simulink model "joystick_control"  (R2012b)
settings: Solver=FixedStepDiscrete  StartTime=0.0  StopTime=inf  FixedStep=0.04  RelTol=1e-3
libraries: etargetslib x14, dspnetwork x11, dspmtrx3 x7, xpcseriallib x7, visionsinks x2, simulink x2, visionstatistics x1, visiontextngfix x1, aerolibanimutils x1, SimulinkExecutionControl x1
settings Model: Creator=Ballistyx  LastModifiedBy=JLEE
settings DataIOCC: SignalLoggingSaveFormat=ModelDataLogs
settings DebuggingCC: MultiTaskDSMMsg=warning  MultiTaskCondExecSysMsg=none  FcnCallInpInsideContextMsg=EnableAllAsWarning  StrictBusMsg=None
settings SFSimCC: SFSimEnableDebug=off
settings RTWCC: IncludeERTFirstTime=on

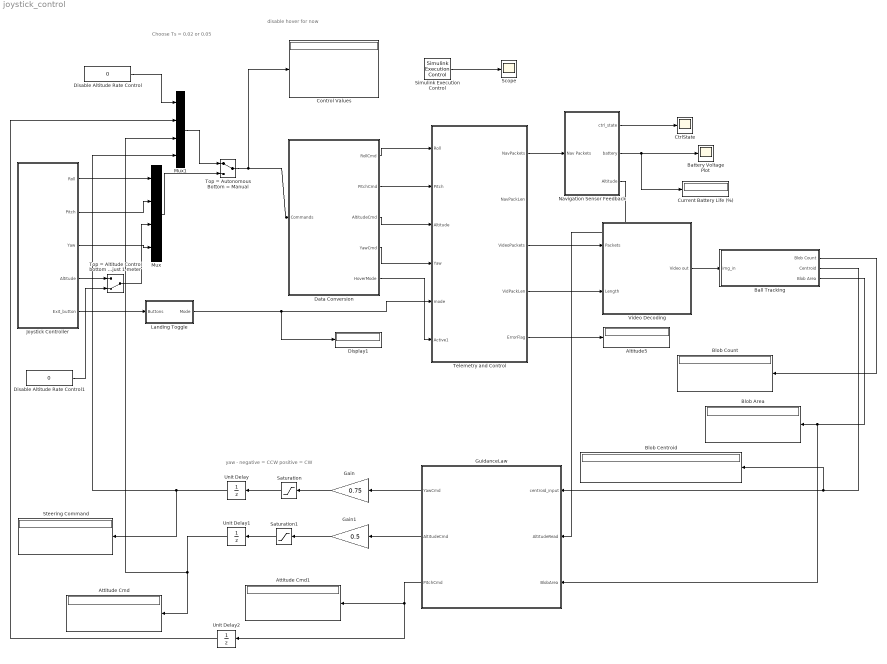
== system joystick_control ==
  note: Choose Ts = 0.02 or 0.05
  note: yaw - negative = CCW
      | positive = CW
  note: disable hover for now
  Altitude5 : Display
  Attitude Cmd : Display
  Attitude Cmd1 : Display
  Ball Tracking : Subsystem
  Battery Voltage Plot : Scope
  Blob Area : Display
  Blob Centroid : Display
  Blob Count : Display
  Control Values : Display
  CtrlState : Scope
      settings: YMin=124518  YMax=137626  SaveName=ScopeData2
  Current Battery Life (%) : Display
  Data Conversion : Subsystem
  Disable Altitude Rate Control : Constant  Value=0
  Disable Altitude Rate Control1 : Constant  Value=0
  Display1 : Display
  Gain : Gain  Gain=0.75
  Gain1 : Gain  Gain=0.5
  GuidanceLaw : Stateflow chart  TreatAsAtomicUnit=on
  Joystick Controller : Subsystem
  Landing Toggle : Subsystem
  Mux : Mux
  Mux1 : Mux
  Navigation Sensor Feedback : Subsystem
  Saturation : Saturate  UpperLimit=1  LowerLimit=-1
  Saturation1 : Saturate  UpperLimit=1  LowerLimit=-1
  Scope : Scope
  Simulink Execution Control : SimulinkExecutionControl/Simulink Execution Control  proc_pri=NORMAL_PRIORITY_CLASS  thread_pri=THREAD_PRIORITY_NORMAL  rt_sim=on  factor=1  ovrrun=Continue execution  Ts=-1
  Steering Command : Display
  Telemetry and Control : Stateflow chart  TreatAsAtomicUnit=on
  Top = Altitude Control bottom = Auto adjust 1-meter : ManualSwitch  CurrentSetting=0
  Top = Autonomous Bottom = Manual : ManualSwitch
  Unit Delay : UnitDelay  SampleTime=-1
  Unit Delay1 : UnitDelay  SampleTime=-1
  Unit Delay2 : UnitDelay  SampleTime=-1
  Video Decoding : Subsystem
  wires:
  Data Conversion/5(HoverMode) -> Telemetry and Control/6(Active1)
  Telemetry and Control/4(VidPackLen) -> Video Decoding/2(Length)
  Telemetry and Control/5(ErrorFlag) -> Altitude5/1
  Data Conversion/2(PitchCmd) -> Telemetry and Control/2(Pitch)
  Data Conversion/1(RollCmd) -> Telemetry and Control/1(Roll)
  Telemetry and Control/3(VideoPackets) -> Video Decoding/1(Packets)
  Simulink Execution Control/1 -> Scope/1
  Disable Altitude Rate Control/1 -> Mux1/1
  Landing Toggle/1(Mode) -> Telemetry and Control/5(mode), Display1/1
  Video Decoding/1(Video out) -> Ball Tracking/1(img_in)
  Ball Tracking/1(Blob Count) -> Blob Count/1
  Telemetry and Control/1(NavPackets) -> Navigation Sensor Feedback/1(Nav Packets)
  Ball Tracking/2(Centroid) -> GuidanceLaw/1(centroid_input), Blob Centroid/1
  Navigation Sensor Feedback/2(battery) -> Current Battery Life (%)/1, Battery Voltage Plot/1
  Navigation Sensor Feedback/1(ctrl_state) -> CtrlState/1
  GuidanceLaw/1(YawCmd) -> Gain/1
  Saturation/1 -> Unit Delay/1
  Unit Delay/1 -> Steering Command/1, Mux1/4
  Gain/1 -> Saturation/1
  Data Conversion/4(YawCmd) -> Telemetry and Control/4(Yaw)
  Data Conversion/3(AltitudeCmd) -> Telemetry and Control/3(Altitude)
  Joystick Controller/5(Exit_button) -> Landing Toggle/1(Buttons)
  Joystick Controller/1(Roll) -> Mux/1
  Joystick Controller/2(Pitch) -> Mux/2
  Joystick Controller/3(Yaw) -> Mux/4
  Mux1/1 -> Top = Autonomous Bottom = Manual/1
  Mux/1 -> Top = Autonomous Bottom = Manual/2
  Top = Autonomous Bottom = Manual/1 -> Data Conversion/1(Commands), Control Values/1
  Ball Tracking/3(Blob Area) -> GuidanceLaw/3(BlobArea), Blob Area/1
  Navigation Sensor Feedback/3(Altitude) -> GuidanceLaw/2(AltitudeRead)
  GuidanceLaw/2(AltitudeCmd) -> Gain1/1
  Gain1/1 -> Saturation1/1
  Unit Delay1/1 -> Mux1/3, Attitude Cmd/1
  Joystick Controller/4(Altitude) -> Top = Altitude Control bottom = Auto adjust 1-meter/1
  Top = Altitude Control bottom = Auto adjust 1-meter/1 -> Mux/3
  Disable Altitude Rate Control1/1 -> Top = Altitude Control bottom = Auto adjust 1-meter/2
  Saturation1/1 -> Unit Delay1/1
  GuidanceLaw/3(PitchCmd) -> Unit Delay2/1, Attitude Cmd1/1
  Unit Delay2/1 -> Mux1/2

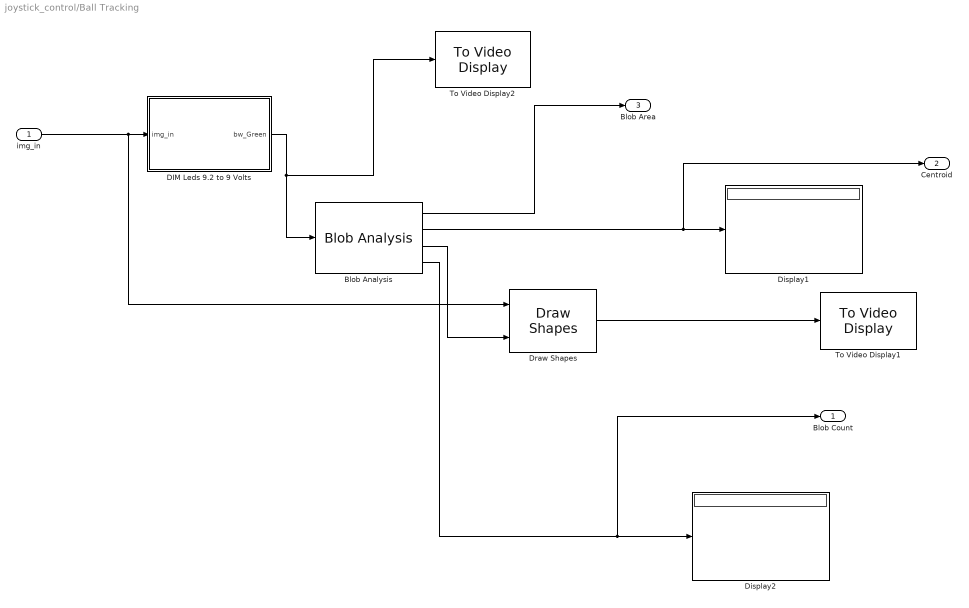
== system joystick_control/Ball Tracking ==
  img_in : Inport
  Blob Analysis : visionstatistics/Blob Analysis  Tag=vipblks_row_conv  area=on  centroid=on  bBox=on  majorAxis=off  minorAxis=off  angle=off  eccentricity=off  equivDiameterSq=off  extent=off  perimeter=off  maxBlobs=1  warnIfNumBlobsExceeded=off  isCount=on  useMinArea=on  minArea=30  useMaxArea=off  maxArea=intmax('uint32')  excludeBorderBlob=on  outDT=double  isOutVarDim=off  isFill=on  fillValues=-1  conn=8  isLabel=off  outputMode=Binary point scaling  outputWordLength=32  outputFracLength=16  firstCoeffMode=Binary point scaling  firstCoeffWordLength=16  firstCoeffFracLength=14  secondCoeffMode=Binary point scaling  secondCoeffWordLength=32  secondCoeffFracLength=16  accumMode=Binary point scaling  accumWordLength=32  accumFracLength=0  prodOutputMode=Binary point scaling  prodOutputWordLength=32  prodOutputFracLength=16  roundingMode=Floor  overflowMode=off
  DIM Leds 9.2 to 9 Volts : MATLAB Function  TreatAsAtomicUnit=on
  Display1 : Display
  Display2 : Display
  Draw Shapes : visiontextngfix/Draw Shapes  shape=Rectangles  fill=off  fillClrSource=Specify via dialog  display=White  intensity=200  color=[200 255 100]  opacity=0.6  viewport=Entire image  antialiasing=off  inType=Obsolete  imagePorts=One multidimensional signal  prodOutputMode=Binary point scaling  prodOutputWordLength=32  prodOutputFracLength=14  memoryMode=Specify word length  memoryWordLength=16  memoryFracLength=15  roundingMode=Floor  overflowMode=off
  To Video Display1 : visionsinks/To Video Display  inputType=Obsolete  imagePorts=One multidimensional signal  OutputDevice=On-screen video monitor  fullScreen=off  videoWindowX=-7  videoWindowY=-15  saveWindowSize=off  videoWindowWidth=1566  videoWindowHeight=1001  dataOrg=Column-major  openAtMdlStart=on  isWindowOpen=on  inputColorFormat=RGB
  To Video Display2 : visionsinks/To Video Display  inputType=Obsolete  imagePorts=One multidimensional signal  OutputDevice=On-screen video monitor  fullScreen=off  videoWindowX=420  videoWindowY=155  saveWindowSize=off  videoWindowWidth=320  videoWindowHeight=240  dataOrg=Column-major  openAtMdlStart=on  isWindowOpen=on  inputColorFormat=RGB
  Blob Count : Outport
  Centroid : Outport  Port=2
  Blob Area : Outport  Port=3
  wires:
  img_in/1 -> DIM Leds 9.2 to 9 Volts/1(img_in), Draw Shapes/1
  DIM Leds 9.2 to 9 Volts/1(bw_Green) -> Blob Analysis/1, To Video Display2/1
  Blob Analysis/3 -> Draw Shapes/2
  Draw Shapes/1 -> To Video Display1/1
  Blob Analysis/2 -> Display1/1, Centroid/1
  Blob Analysis/4 -> Display2/1, Blob Count/1
  Blob Analysis/1 -> Blob Area/1

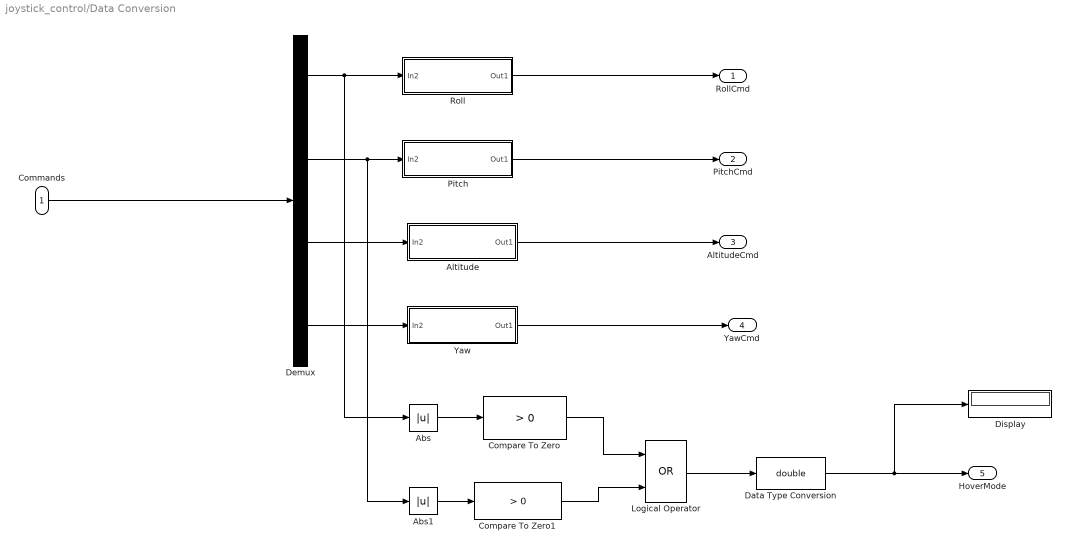
== system joystick_control/Data Conversion ==
  Commands : Inport
  Abs : Abs
  Abs1 : Abs
  Altitude : Subsystem
  Compare To Zero : simulink/Logic and Bit Operations/Compare To Zero  relop=>  OutDataTypeStr=uint8
  Compare To Zero1 : simulink/Logic and Bit Operations/Compare To Zero  relop=>  OutDataTypeStr=uint8
  Data Type Conversion : DataTypeConversion  OutDataTypeStr=double
  Demux : Demux
  Display : Display
  Logical Operator : Logic  Operator=OR  AllPortsSameDT=off  OutDataTypeStr=boolean
  Pitch : Subsystem
  Roll : Subsystem
  Yaw : Subsystem
  RollCmd : Outport
  PitchCmd : Outport  Port=2
  AltitudeCmd : Outport  Port=3
  YawCmd : Outport  Port=4
  HoverMode : Outport  Port=5
  wires:
  Demux/1 -> Roll/1(In2), Abs/1
  Demux/2 -> Pitch/1(In2), Abs1/1
  Demux/3 -> Altitude/1(In2)
  Demux/4 -> Yaw/1(In2)
  Commands/1 -> Demux/1
  Roll/1(Out1) -> RollCmd/1
  Pitch/1(Out1) -> PitchCmd/1
  Altitude/1(Out1) -> AltitudeCmd/1
  Yaw/1(Out1) -> YawCmd/1
  Compare To Zero/1 -> Logical Operator/1
  Compare To Zero1/1 -> Logical Operator/2
  Logical Operator/1 -> Data Type Conversion/1
  Data Type Conversion/1 -> HoverMode/1, Display/1
  Abs/1 -> Compare To Zero/1
  Abs1/1 -> Compare To Zero1/1

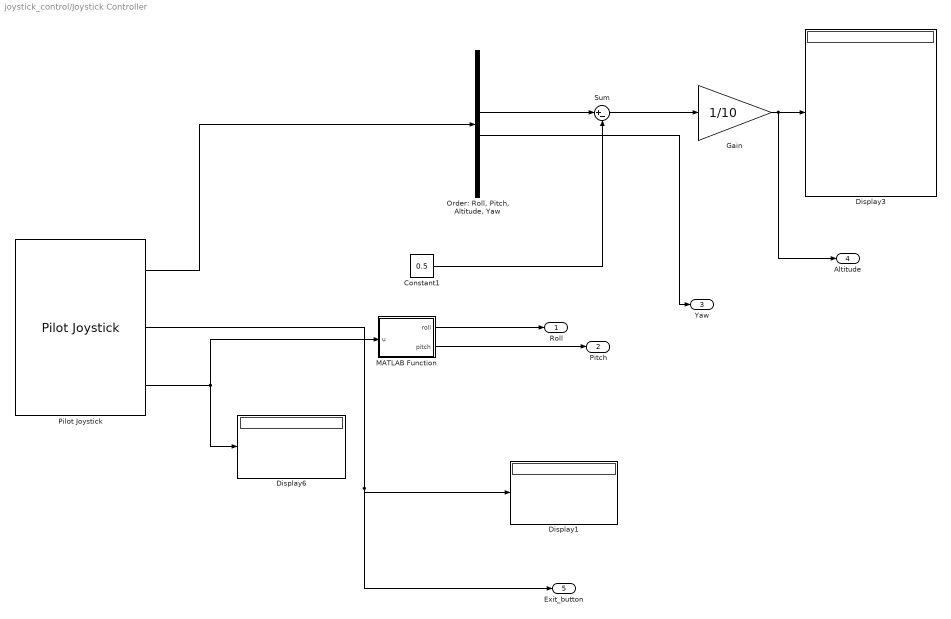
== system joystick_control/Joystick Controller ==
  Constant1 : Constant  Value=0.5
  Display1 : Display
  Display3 : Display
  Display6 : Display
  Gain : Gain  Gain=1/10
  MATLAB Function : MATLAB Function  TreatAsAtomicUnit=on
  "Order: Roll, Pitch, Altitude, Yaw" : Demux  Outputs=6
  Pilot Joystick : aerolibanimutils/Pilot Joystick  JoystickID=Joystick1  OutputConfiguration=AllOutputs  SampleTime=-1
  Sum : Sum  Inputs=|+-
  Roll : Outport
  Pitch : Outport  Port=2
  Yaw : Outport  Port=3
  Altitude : Outport  Port=4
  Exit_button : Outport  Port=5
  wires:
  Pilot Joystick/1 -> "Order: Roll, Pitch, Altitude, Yaw"/1
  Pilot Joystick/3 -> Display6/1, MATLAB Function/1(u)
  "Order: Roll, Pitch, Altitude, Yaw"/3 -> Sum/1
  Constant1/1 -> Sum/2
  Sum/1 -> Gain/1
  MATLAB Function/1(roll) -> Roll/1
  MATLAB Function/2(pitch) -> Pitch/1
  Gain/1 -> Display3/1, Altitude/1
  "Order: Roll, Pitch, Altitude, Yaw"/4 -> Yaw/1
  Pilot Joystick/2 -> Display1/1, Exit_button/1

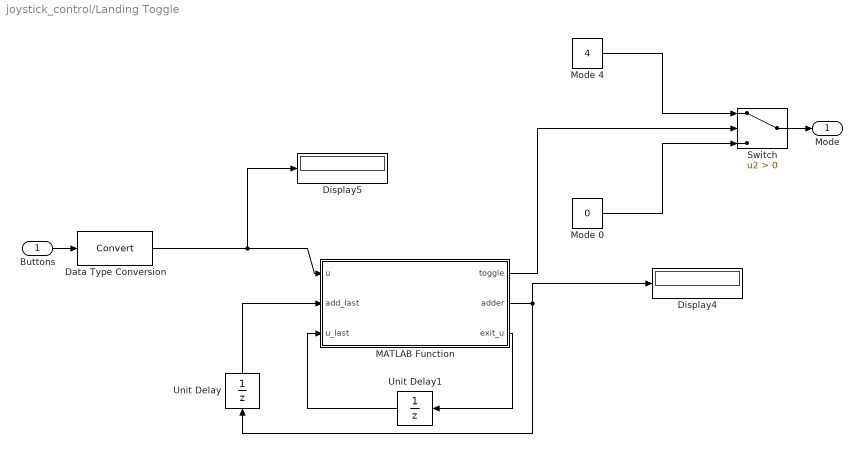
== system joystick_control/Landing Toggle ==
  Buttons : Inport
  Data Type Conversion : DataTypeConversion
  Display4 : Display
  Display5 : Display
  MATLAB Function : MATLAB Function  TreatAsAtomicUnit=on
  Mode 0 : Constant  Value=0
  Mode 4 : Constant  Value=4
  Switch : Switch  Criteria=u2 > Threshold
  Unit Delay : UnitDelay  SampleTime=-1
  Unit Delay1 : UnitDelay  SampleTime=-1
  Mode : Outport
  wires:
  Unit Delay/1 -> MATLAB Function/2(add_last)
  MATLAB Function/2(adder) -> Display4/1, Unit Delay/1
  MATLAB Function/3(exit_u) -> Unit Delay1/1
  Unit Delay1/1 -> MATLAB Function/3(u_last)
  Data Type Conversion/1 -> MATLAB Function/1(u), Display5/1
  MATLAB Function/1(toggle) -> Switch/2
  Mode 4/1 -> Switch/1
  Mode 0/1 -> Switch/3
  Switch/1 -> Mode/1
  Buttons/1 -> Data Type Conversion/1

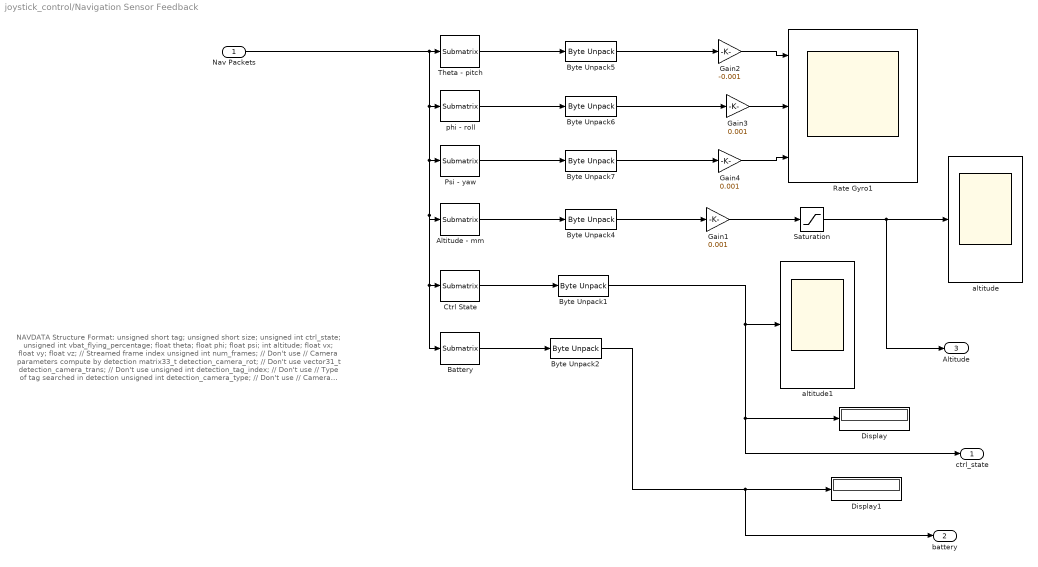
== system joystick_control/Navigation Sensor Feedback ==
  note: NAVDATA Structure Format:
      |
      |         unsigned short tag;
      |         unsigned short size;
      |         unsigned int   ctrl_state;
      |         unsigned int   vbat_flying_percentage;
      |         float          theta;
      |         float          phi;
      |         float          psi;
      |         int            altitude;
      |         float          vx;
      |         float          vy;
      |         float          vz;
      |
      |         // Streamed frame index
      |         unsigned int num_frames;                // Don't use
      |
      |         // Camera parameters compute by detection
      |         matrix33_t   detection_camera_rot;      // Don't use
      |         vector31_t   detection_camera_trans;    // Don't use
      |         unsigned int detection_tag_index;       // Don't use
      |
      |         // Type of tag searched in detection
      |         unsigned int detection_camera_type;     // Don't use
      |
      |         // Camera parameters compute by drone
      |         matrix33_t drone_camera_rot;            // Don't use
      |         vector31_t drone_camera_trans;          // Don't use
  Nav Packets : Inport
  Altitude - mm : dspmtrx3/Submatrix  RowSpan=Range of rows  RowStartMode=Index  RowStartIndex=41  RowEndMode=Index  RowEndIndex=44  ColSpan=All columns  ColStartMode=Index  ColStartIndex=4  ColEndMode=Index  ColEndIndex=4
  Battery : dspmtrx3/Submatrix  RowSpan=Range of rows  RowStartMode=Index  RowStartIndex=25  RowEndMode=Index  RowEndIndex=28  ColSpan=All columns  ColStartMode=Index  ColStartIndex=4  ColEndMode=Index  ColEndIndex=4
  Byte Unpack1 : etargetslib/Byte Unpack  dimensions={[1]}  datatypes={'uint32'}  byteAlign=1
  Byte Unpack2 : etargetslib/Byte Unpack  dimensions={[1]}  datatypes={'uint32'}  byteAlign=1
  Byte Unpack4 : etargetslib/Byte Unpack  dimensions={[1]}  datatypes={'uint32'}  byteAlign=1
  Byte Unpack5 : etargetslib/Byte Unpack  dimensions={[1]}  datatypes={'single'}  byteAlign=1
  Byte Unpack6 : etargetslib/Byte Unpack  dimensions={[1]}  datatypes={'single'}  byteAlign=1
  Byte Unpack7 : etargetslib/Byte Unpack  dimensions={[1]}  datatypes={'single'}  byteAlign=1
  Ctrl State : dspmtrx3/Submatrix  RowSpan=Range of rows  RowStartMode=Index  RowStartIndex=21  RowEndMode=Index  RowEndIndex=24  ColSpan=All columns  ColStartMode=Index  ColStartIndex=4  ColEndMode=Index  ColEndIndex=4
  Display : Display
  Display1 : Display
  Gain1 : Gain  Gain=0.001  OutDataTypeStr=double
  Gain2 : Gain  Gain=-0.001
  Gain3 : Gain  Gain=0.001
  Gain4 : Gain  Gain=0.001
  Psi - yaw : dspmtrx3/Submatrix  RowSpan=Range of rows  RowStartMode=Index  RowStartIndex=37  RowEndMode=Index  RowEndIndex=40  ColSpan=All columns  ColStartMode=Index  ColStartIndex=4  ColEndMode=Index  ColEndIndex=4
  Rate Gyro1 : Scope  NumInputPorts=3
      settings: TimeRange=18  YMin=-0.75~2.935~53.5  YMax=0~3~60  SaveName=NavData_Simulink1
  Saturation : Saturate  UpperLimit=10  LowerLimit=0  OutDataTypeStr=Inherit: Inherit via back propagation
  Theta - pitch : dspmtrx3/Submatrix  RowSpan=Range of rows  RowStartMode=Index  RowStartIndex=29  RowEndMode=Index  RowEndIndex=32  ColSpan=All columns  ColStartMode=Index  ColStartIndex=4  ColEndMode=Index  ColEndIndex=4
  altitude : Scope
      settings: YMin=0.242  YMax=0.24305  SaveName=NavData_Simulink
  altitude1 : Scope
      settings: YMin=0.242  YMax=0.24305  SaveName=NavData_Simulink2
  phi - roll : dspmtrx3/Submatrix  RowSpan=Range of rows  RowStartMode=Index  RowStartIndex=33  RowEndMode=Index  RowEndIndex=36  ColSpan=All columns  ColStartMode=Index  ColStartIndex=4  ColEndMode=Index  ColEndIndex=4
  ctrl_state : Outport
  battery : Outport  Port=2
  Altitude : Outport  Port=3
  wires:
  Altitude - mm/1 -> Byte Unpack4/1
  Theta - pitch/1 -> Byte Unpack5/1
  phi - roll/1 -> Byte Unpack6/1
  Psi - yaw/1 -> Byte Unpack7/1
  Byte Unpack5/1 -> Gain2/1
  Byte Unpack6/1 -> Gain3/1
  Byte Unpack7/1 -> Gain4/1
  Byte Unpack4/1 -> Gain1/1
  Gain1/1 -> Saturation/1
  Gain2/1 -> Rate Gyro1/1
  Gain3/1 -> Rate Gyro1/2
  Gain4/1 -> Rate Gyro1/3
  Nav Packets/1 -> Psi - yaw/1, Altitude - mm/1, Ctrl State/1, Battery/1, phi - roll/1, Theta - pitch/1
  Saturation/1 -> altitude/1, Altitude/1
  Ctrl State/1 -> Byte Unpack1/1
  Byte Unpack1/1 -> altitude1/1, Display/1, ctrl_state/1
  Battery/1 -> Byte Unpack2/1
  Byte Unpack2/1 -> Display1/1, battery/1

== system joystick_control/Telemetry and Control/SetVideo ==
  DataStamp : Inport
  f : TriggerPort  TriggerType=function-call
      settings: CopyFcn=Stateflow.SLINSF.SimulinkMan.removeBlockPreDeleteFcn  PreDeleteFcn=Stateflow.SLINSF.SimulinkMan.unsafePredeleteFcn
  ASCII Encode 1 : xpcseriallib/ASCII Encode   format="AT*CONFIG=%d,\\\"video:video_channel\\\",\\\"0\\\"\\r"  nvars=1  maxlength=44  vartypes={ 'uint32' }
  UDP Send : dspnetwork/UDP Send  remoteURL='192.168.1.1'  remotePort=5556  localURL='0.0.0.0'  localPortSource=Specify via dialog  localPort=5556  sampletime=-1  separateLengthPort=0
  wires:
  DataStamp/1 -> ASCII Encode 1/1
  ASCII Encode 1/1 -> UDP Send/1

== system joystick_control/Telemetry and Control/StartNavDemo ==
  note: Enable navdatademo
  DataStamp : Inport
  f : TriggerPort  TriggerType=function-call
      settings: CopyFcn=Stateflow.SLINSF.SimulinkMan.removeBlockPreDeleteFcn  PreDeleteFcn=Stateflow.SLINSF.SimulinkMan.unsafePredeleteFcn
  ASCII Encode 2 : xpcseriallib/ASCII Encode   format="AT*CONFIG=%d,\\\"general:navdata_demo\\\",\\\"TRUE\\\"\\r"  nvars=1  maxlength=43  vartypes={ 'uint32' }
  UDP Send1 : dspnetwork/UDP Send  remoteURL='192.168.1.1'  remotePort=5556  localURL='0.0.0.0'  localPortSource=Specify via dialog  localPort=5556  sampletime=-1  separateLengthPort=0
  wires:
  DataStamp/1 -> ASCII Encode 2/1
  ASCII Encode 2/1 -> UDP Send1/1

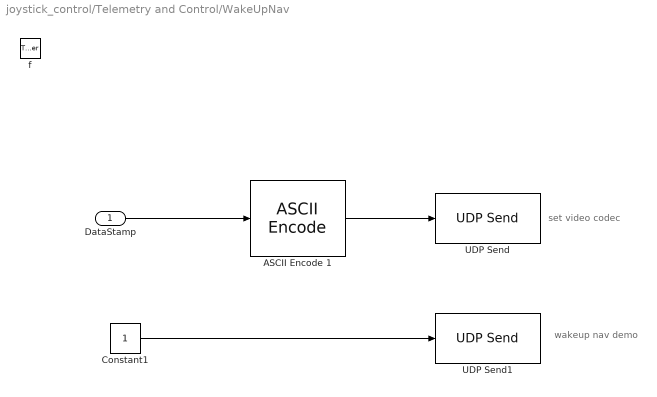
== system joystick_control/Telemetry and Control/WakeUpNav ==
  note: set video codec
  note: wakeup nav demo
  DataStamp : Inport
  f : TriggerPort  TriggerType=function-call
      settings: CopyFcn=Stateflow.SLINSF.SimulinkMan.removeBlockPreDeleteFcn  PreDeleteFcn=Stateflow.SLINSF.SimulinkMan.unsafePredeleteFcn
  ASCII Encode 1 : xpcseriallib/ASCII Encode   format="AT*CONFIG=%d,\\\"video:video_codec\\\",\\\"32\\\"\\r"  nvars=1  maxlength=44  vartypes={ 'uint32' }
  Constant1 : Constant  OutDataTypeStr=uint8  SampleTime=-1
  UDP Send : dspnetwork/UDP Send  remoteURL='192.168.1.1'  remotePort=5556  localURL='0.0.0.0'  localPortSource=Specify via dialog  localPort=5556  sampletime=-1  separateLengthPort=0
  UDP Send1 : dspnetwork/UDP Send  remoteURL='192.168.1.1'  remotePort=5554  localURL='0.0.0.0'  localPortSource=Specify via dialog  localPort=5554  sampletime=-1  separateLengthPort=0
  wires:
  DataStamp/1 -> ASCII Encode 1/1
  Constant1/1 -> UDP Send1/1
  ASCII Encode 1/1 -> UDP Send/1

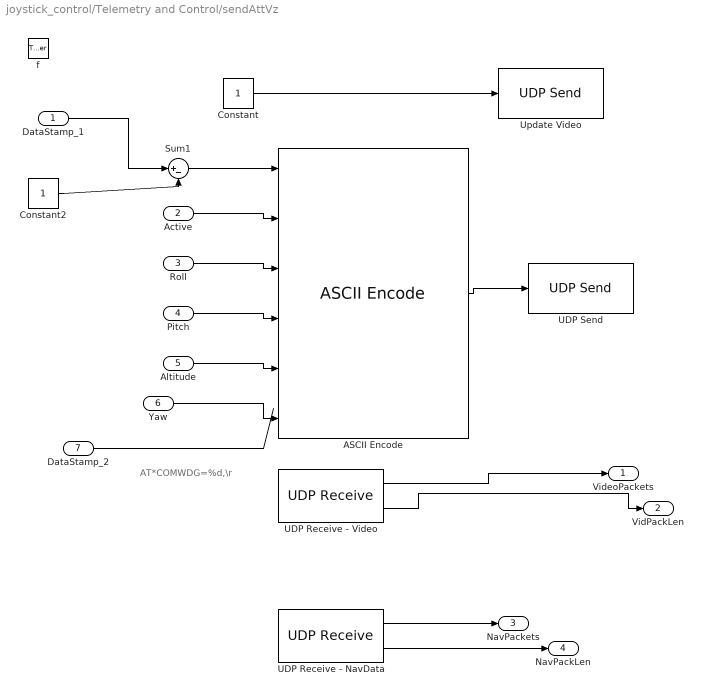
== system joystick_control/Telemetry and Control/sendAttVz ==
  note: AT*COMWDG=%d,\r
  DataStamp_1 : Inport
  Active : Inport  Port=2
  Roll : Inport  Port=3
  Pitch : Inport  Port=4
  Altitude : Inport  Port=5
  Yaw : Inport  Port=6
  DataStamp_2 : Inport  Port=7
  f : TriggerPort  TriggerType=function-call
      settings: CopyFcn=Stateflow.SLINSF.SimulinkMan.removeBlockPreDeleteFcn  PreDeleteFcn=Stateflow.SLINSF.SimulinkMan.unsafePredeleteFcn
  "ASCII Encode " : xpcseriallib/ASCII Encode   format=AT*PCMD=%d,%d,%d,%d,%d,%d\r  nvars=6  maxlength=128  vartypes={ 'double' }
  Constant : Constant  Priority=12  OutDataTypeStr=uint8  SampleTime=-1
  Constant2 : Constant
  Sum1 : Sum  Inputs=|+-
  UDP Receive - NavData : dspnetwork/UDP Receive  Priority=15  localURL='0.0.0.0'  localPort=5554  remoteURL='192.168.1.1'  remotePort=-1  recvBufferSize=500  dims=500  signalDatatype=uint8  isVarSize=off  showBlockingTime=off  blockingTime=0  sampletime=-1
  UDP Receive - Video : dspnetwork/UDP Receive  Priority=16  localURL='0.0.0.0'  localPort=5555  remoteURL='192.168.1.1'  remotePort=-1  recvBufferSize=40000*2  dims=40000  signalDatatype=uint8  isVarSize=off  showBlockingTime=off  blockingTime=0  sampletime=-1
  UDP Send : dspnetwork/UDP Send  Priority=11  remoteURL='192.168.1.1'  remotePort=5556  localURL='0.0.0.0'  localPortSource=Specify via dialog  localPort=5556  sampletime=-1  separateLengthPort=0
  Update Video : dspnetwork/UDP Send  Priority=10  remoteURL='192.168.1.1'  remotePort=5555  localURL='0.0.0.0'  localPortSource=Specify via dialog  localPort=5555  sampletime=-1  separateLengthPort=0
  VideoPackets : Outport
  VidPackLen : Outport  Port=2  OutDataTypeStr=uint16
  NavPackets : Outport  Port=3
  NavPackLen : Outport  Port=4
  wires:
  Active/1 -> "ASCII Encode "/2
  Roll/1 -> "ASCII Encode "/3
  Pitch/1 -> "ASCII Encode "/4
  Altitude/1 -> "ASCII Encode "/5
  Yaw/1 -> "ASCII Encode "/6
  DataStamp_2/1 -> ?
  DataStamp_1/1 -> Sum1/1
  Sum1/1 -> "ASCII Encode "/1
  Constant2/1 -> Sum1/2
  "ASCII Encode "/1 -> UDP Send/1
  Constant/1 -> Update Video/1
  UDP Receive - Video/2 -> VidPackLen/1
  UDP Receive - NavData/2 -> NavPackLen/1
  UDP Receive - Video/1 -> VideoPackets/1
  UDP Receive - NavData/1 -> NavPackets/1

== system joystick_control/Telemetry and Control/sendLand ==
  In1 : Inport
  f : TriggerPort  TriggerType=function-call
      settings: CopyFcn=Stateflow.SLINSF.SimulinkMan.removeBlockPreDeleteFcn  PreDeleteFcn=Stateflow.SLINSF.SimulinkMan.unsafePredeleteFcn
  "ASCII Encode " : xpcseriallib/ASCII Encode   format=AT*REF=%d,290717696\r  nvars=1  maxlength=128  vartypes={ 'double' }
  UDP Send : dspnetwork/UDP Send  remoteURL='192.168.1.1'  remotePort=5556  localURL='0.0.0.0'  localPortSource=Specify via dialog  localPort=5556  sampletime=-1  separateLengthPort=0
  wires:
  "ASCII Encode "/1 -> UDP Send/1
  In1/1 -> "ASCII Encode "/1

== system joystick_control/Telemetry and Control/sendTrim ==
  DataStamp : Inport
  f : TriggerPort  TriggerType=function-call
      settings: CopyFcn=Stateflow.SLINSF.SimulinkMan.removeBlockPreDeleteFcn  PreDeleteFcn=Stateflow.SLINSF.SimulinkMan.unsafePredeleteFcn
  "ASCII Encode " : xpcseriallib/ASCII Encode   format=AT*FTRIM=%d,\r  nvars=1  maxlength=128  vartypes={ 'double' }
  UDP Send : dspnetwork/UDP Send  remoteURL='192.168.1.1'  remotePort=5556  localURL='0.0.0.0'  localPortSource=Specify via dialog  localPort=5556  sampletime=-1  separateLengthPort=0
  wires:
  DataStamp/1 -> "ASCII Encode "/1
  "ASCII Encode "/1 -> UDP Send/1

== system joystick_control/Telemetry and Control/startHover ==
  note: disable hover for now
  DataStamp : Inport
  f : TriggerPort  TriggerType=function-call
      settings: CopyFcn=Stateflow.SLINSF.SimulinkMan.removeBlockPreDeleteFcn  PreDeleteFcn=Stateflow.SLINSF.SimulinkMan.unsafePredeleteFcn
  "ASCII Encode " : xpcseriallib/ASCII Encode   format=AT*REF=%d,290718208\r  nvars=1  maxlength=128  vartypes={ 'double' }
  UDP Send : dspnetwork/UDP Send  remoteURL='192.168.1.1'  remotePort=5556  localURL='0.0.0.0'  localPortSource=Specify via dialog  localPort=5556  sampletime=-1  separateLengthPort=0
  wires:
  DataStamp/1 -> "ASCII Encode "/1
  "ASCII Encode "/1 -> UDP Send/1

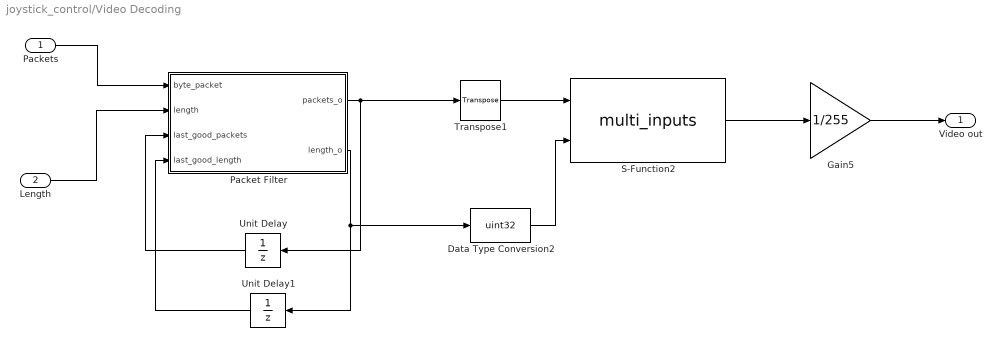
== system joystick_control/Video Decoding ==
  Packets : Inport
  Length : Inport  Port=2
  Data Type Conversion2 : DataTypeConversion  OutDataTypeStr=uint32
  Gain5 : Gain  Gain=1/255
  Packet Filter : MATLAB Function  TreatAsAtomicUnit=on
  S-Function2 : S-Function  FunctionName=multi_inputs  EnableBusSupport=off
  Transpose1 : dspmtrx3/Transpose  Hermitian=off  overflowFlag=off
  Unit Delay : UnitDelay  SampleTime=-1
  Unit Delay1 : UnitDelay  SampleTime=-1
  Video out : Outport
  wires:
  Data Type Conversion2/1 -> S-Function2/2
  S-Function2/1 -> Gain5/1
  Transpose1/1 -> S-Function2/1
  Packet Filter/1(packets_o) -> Unit Delay/1, Transpose1/1
  Unit Delay/1 -> Packet Filter/3(last_good_packets)
  Packet Filter/2(length_o) -> Unit Delay1/1, Data Type Conversion2/1
  Unit Delay1/1 -> Packet Filter/4(last_good_length)
  Packets/1 -> Packet Filter/1(byte_packet)
  Length/1 -> Packet Filter/2(length)
  Gain5/1 -> Video out/1

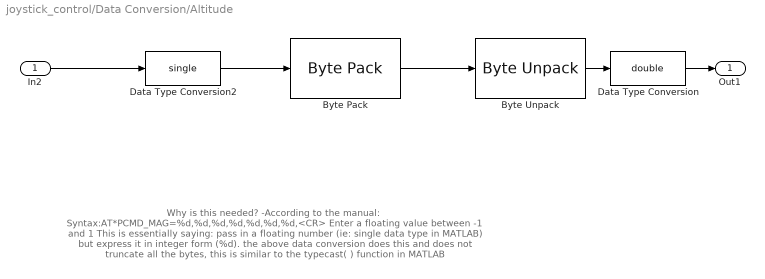
== system joystick_control/Data Conversion/Altitude ==
  note: Why is this needed?
      | -According to the manual:
      |
      | Syntax:AT*PCMD_MAG=%d,%d,%d,%d,%d,%d,%d,<CR>
      | Enter a floating value between -1 and 1
      |
      | This is essentially saying: pass in a floating number (ie: single data type in MATLAB) but express it in integer form (%d).
      | the above data conversion does this and does not truncate all the bytes, this is similar to the typecast( ) function in MATLAB
  In2 : Inport
  Byte Pack : etargetslib/Byte Pack  datatypes={'single'}  byteAlign=1
  Byte Unpack : etargetslib/Byte Unpack  dimensions={[1]}  datatypes={'int32'}  byteAlign=1
  Data Type Conversion : DataTypeConversion  OutDataTypeStr=double
  Data Type Conversion2 : DataTypeConversion  OutDataTypeStr=single
  Out1 : Outport
  wires:
  Byte Pack/1 -> Byte Unpack/1
  Byte Unpack/1 -> Data Type Conversion/1
  In2/1 -> Data Type Conversion2/1
  Data Type Conversion2/1 -> Byte Pack/1
  Data Type Conversion/1 -> Out1/1

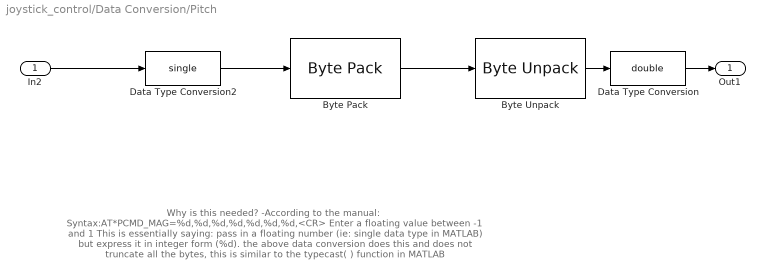
== system joystick_control/Data Conversion/Pitch ==
  note: Why is this needed?
      | -According to the manual:
      |
      | Syntax:AT*PCMD_MAG=%d,%d,%d,%d,%d,%d,%d,<CR>
      | Enter a floating value between -1 and 1
      |
      | This is essentially saying: pass in a floating number (ie: single data type in MATLAB) but express it in integer form (%d).
      | the above data conversion does this and does not truncate all the bytes, this is similar to the typecast( ) function in MATLAB
  In2 : Inport
  Byte Pack : etargetslib/Byte Pack  datatypes={'single'}  byteAlign=1
  Byte Unpack : etargetslib/Byte Unpack  dimensions={[1]}  datatypes={'int32'}  byteAlign=1
  Data Type Conversion : DataTypeConversion  OutDataTypeStr=double
  Data Type Conversion2 : DataTypeConversion  OutDataTypeStr=single
  Out1 : Outport
  wires:
  Byte Pack/1 -> Byte Unpack/1
  Byte Unpack/1 -> Data Type Conversion/1
  In2/1 -> Data Type Conversion2/1
  Data Type Conversion2/1 -> Byte Pack/1
  Data Type Conversion/1 -> Out1/1

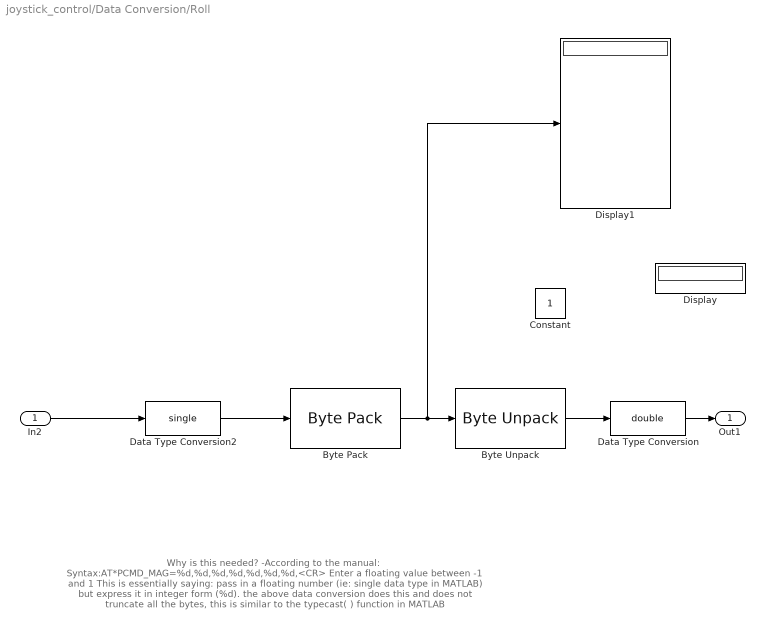
== system joystick_control/Data Conversion/Roll ==
  note: Why is this needed?
      | -According to the manual:
      |
      | Syntax:AT*PCMD_MAG=%d,%d,%d,%d,%d,%d,%d,<CR>
      | Enter a floating value between -1 and 1
      |
      | This is essentially saying: pass in a floating number (ie: single data type in MATLAB) but express it in integer form (%d).
      | the above data conversion does this and does not truncate all the bytes, this is similar to the typecast( ) function in MATLAB
  In2 : Inport
  Byte Pack : etargetslib/Byte Pack  datatypes={'single'}  byteAlign=1
  Byte Unpack : etargetslib/Byte Unpack  dimensions={[1]}  datatypes={'int32'}  byteAlign=1
  Constant : Constant
  Data Type Conversion : DataTypeConversion  OutDataTypeStr=double
  Data Type Conversion2 : DataTypeConversion  OutDataTypeStr=single
  Display : Display
  Display1 : Display
  Out1 : Outport
  wires:
  In2/1 -> Data Type Conversion2/1
  Data Type Conversion2/1 -> Byte Pack/1
  Data Type Conversion/1 -> Out1/1
  Byte Pack/1 -> Byte Unpack/1, Display1/1
  Byte Unpack/1 -> Data Type Conversion/1
  ? -> Display/1

== system joystick_control/Data Conversion/Yaw ==
  note: Why is this needed?
      | -According to the manual:
      |
      | Syntax:AT*PCMD_MAG=%d,%d,%d,%d,%d,%d,%d,<CR>
      | Enter a floating value between -1 and 1
      |
      | This is essentially saying: pass in a floating number (ie: single data type in MATLAB) but express it in integer form (%d).
      | the above data conversion does this and does not truncate all the bytes, this is similar to the typecast( ) function in MATLAB
  In2 : Inport
  Byte Pack : etargetslib/Byte Pack  datatypes={'single'}  byteAlign=1
  Byte Unpack : etargetslib/Byte Unpack  dimensions={[1]}  datatypes={'int32'}  byteAlign=1
  Data Type Conversion : DataTypeConversion  OutDataTypeStr=double
  Data Type Conversion2 : DataTypeConversion  OutDataTypeStr=single
  Out1 : Outport
  wires:
  Byte Pack/1 -> Byte Unpack/1
  Byte Unpack/1 -> Data Type Conversion/1
  In2/1 -> Data Type Conversion2/1
  Data Type Conversion2/1 -> Byte Pack/1
  Data Type Conversion/1 -> Out1/1

== matlab function joystick_control/Video Decoding/Packet Filter ==
  data: byte_packet input; packets_o output; length input uint16; last_good_packets input; length_o output uint16; last_good_length input
function [packets_o,length_o] = fcn(byte_packet,length,last_good_packets,last_good_length)
%#codegen

if length == 0
    packets_o = last_good_packets;
    length_o = last_good_length;
else
    packets_o = byte_packet; 
    length_o = length;
end

== matlab function joystick_control/Landing Toggle/MATLAB Function ==
  data: toggle output; u input; add_last input; adder output; exit_u output double; u_last input
function [toggle,adder,exit_u] = fcn(u,add_last,u_last)
%#codegen

% if u ~= last_u
% y = 1;
% else
% y = 0;    
% end
% 

if (u==64 & (u_last == 0))
    
   adder = add_last + 1;
%     exit_u = u;
else
    adder = add_last;
%     exit_u = u;
end

 exit_u = u;
 
 toggle=mod(adder,2);

% y = u;

== stateflow chart joystick_control/GuidanceLaw ==
  state Steering_Law [parallel]
    settings: executionOrder=1
    state NoBall
      YawCmd = 0;
    state WithinFOV_x
      YawCmd = 0;
    state Steering
      du: YawCmd = SteerYaw(centroid_input);
    (default) -> (junction 131)
    (junction 131) -> Steering_Law.NoBall : {i=0;
        | InitiateVariables_x();}
    Steering -> Steering_Law.NoBall [order 2] : [centroid_input[0] == -1 ]
    Steering_Law.NoBall -> WithinFOV_x : [centroid_input[0] != -1  ]
        | {i = i + 1;}
    WithinFOV_x -> Steering [order 1] : [ (centroid_input[0]<SearchField_left || centroid_input[0]>SearchField_right) && centroid_input[0] != -1]
        | {i = i + 1;}
    WithinFOV_x -> Steering_Law.NoBall [order 2] : [centroid_input[0] == -1 ]
        | {i = i + 1;}
    Steering -> WithinFOV_x [order 1] : [ (centroid_input[0]>=SearchField_left && centroid_input[0]<=SearchField_right) && centroid_input[0] != -1]
        | {i = i + 1;}
  state Pitch_Cmd [parallel]
    settings: executionOrder=3
    state NoBall
      PitchCmd = 0;
    state StopFollowing
      PitchCmd = 0;
    state FollowBall
      PitchCmd = -0.05;
    (default) -> (junction 183)
    (junction 183) -> Pitch_Cmd.NoBall : {i=0;
        | PitchInitiate();}
    StopFollowing -> Pitch_Cmd.NoBall [order 1] : [BlobArea == -1]
    Pitch_Cmd.NoBall -> StopFollowing : [BlobArea != -1]
    FollowBall -> StopFollowing : [BlobArea>BlobAreaThresholdLo || YawCmd!=0  || YawCmd!=0]
    StopFollowing -> FollowBall [order 2] : [BlobArea<=BlobAreaThresholdLo && YawCmd==0 && AltitudeCmd==0]
  state Altitude_Cmd [parallel]
    settings: executionOrder=2
    state NoBall
      AltitudeCmd  = 0;
    state WithinFOV_y
      AltitudeCmd = 0;
    state Altitude_Correct
      du: AltitudeCmd = ChangeAltitude(centroid_input);
    (default) -> (junction 158)
    (junction 158) -> Altitude_Cmd.NoBall : {i=0;
        | InitiateVariables_y();}
    Altitude_Correct -> Altitude_Cmd.NoBall [order 1] : [centroid_input[1] == -1 ]
    WithinFOV_y -> Altitude_Correct [order 2] : [ (centroid_input[1]>=SearchField_Bottom || centroid_input[1]<=SearchField_Top) && centroid_input[1] != -1]
        | {i = i + 1;}
    Altitude_Cmd.NoBall -> WithinFOV_y : [centroid_input[1] != -1  ]
        | {i = i + 1;}
    WithinFOV_y -> Altitude_Cmd.NoBall [order 1] : [centroid_input[1] == -1  ]
        | {i = i + 1;}
    Altitude_Correct -> WithinFOV_y [order 2] : [ (centroid_input[1]<SearchField_Bottom && centroid_input[1]>SearchField_Top) && centroid_input[1] != -1]
        | {i = i + 1;}
  data: YawCmd function_output double size=1; centroid_input function_input double size=2; AltitudeCmd function_output double size=1; centroid function_input double size=2; centroid_input input double size=2; Roll local double; Pitch local double; YawCmd output double =0; AltitudeRead input double size=1; i local double; SearchField_left local double; SearchField_right local double; AltitudeCmd output double; SearchField_Bottom local double; SearchField_Top local double; BlobAreaThresholdHi local double; PitchCmd output double; BlobArea input int32; BlobAreaThresholdLo local double
  function InitiateVariables_x:
    | function InitiateVariables_x
    | %used to define search thresholds
    | SearchField_left = 130;
    | SearchField_right = 190;
  function YawCmd = SteerYaw(centroid_input):
    | function YawCmd = SteerYaw(centroid_input)
    | 
    | img_row_center = 160;
    | gain = 1/160; %will use max speed if ball is at extremes
    | error = centroid_input(1) - img_row_center;
    | 
    | %positive error, ball is on the right side, turn CCW (positive rotation)
    | %negative error, ball is on the left side, turn CW (negative rotatoin)
    | 
    | YawCmd = 1*error*gain;
    | end
  function PitchInitiate:
    | function PitchInitiate
    | 
    | BlobAreaThresholdHi = 400;
    | BlobAreaThresholdLo = 300;
    | end
  function InitiateVariables_y:
    | function InitiateVariables_y
    | %used to define search thresholds
    | SearchField_Top = 100;
    | SearchField_Bottom = 140;
  function AltitudeCmd = ChangeAltitude(centroid):
    | function AltitudeCmd = ChangeAltitude(centroid)
    | 
    | img_row_center = 120;
    | gain = 1/120; %will use max speed if ball is at extremes
    | error = centroid(2) - img_row_center;
    | 
    | %positive error, ball is on the right side, turn CCW (positive rotation)
    | %negative error, ball is on the left side, turn CW (negative rotatoin)
    | 
    | AltitudeCmd = -1*error*gain;
    | end

== matlab function joystick_control/Joystick Controller/MATLAB Function ==
  data: u input; roll output; pitch output
function [roll,pitch] = fcn(u)
%#codegen

if u == 0
    roll  = 0;
    pitch = -0.2;
%     yaw   = 
elseif u == 180
    roll  = 0;
    pitch = 0.2;
%     yaw   = 
    
elseif u == 90
    roll  = 0.2;
    pitch = 0;
%     yaw   = 
    
elseif u == 270
    roll  = -0.2;
    pitch = 0;
%     yaw   = 
else
    
    roll  = 0;
    pitch = 0;
%     yaw   = 0;
    
end

== stateflow chart joystick_control/Telemetry and Control ==
  state ExecuteTrimCmd_State
    entry:ErrorFlag = 0;
    during: sendTrim(i)
  state ModeSelector
  state sendTrim(DataStamp) [function]
  state WakeUpNavVideo_State
    entry:ErrorFlag = 0;
    during: WakeUpNav(i)
  state WakeUpNav(DataStamp) [function]
  state StartNavDemo_State
    entry:ErrorFlag = 0;
    during: StartNavDemo(i)
  state StartNavDemo(DataStamp) [function]
  state SetVideoChannel_State
    entry:ErrorFlag = 0;
    during: SetVideo(i)
  state SetVideo(DataStamp) [function]
  state BeginHover_State
    entry:ErrorFlag = 0;
    during: startHover(i)
  state startHover(DataStamp) [function]
  state RunMotor6
    entry:ErrorFlag = 0;
    during: sendLand(i)
  state sendLand(In1) [function]
  state Control_State
    entry:ErrorFlag = 0;
    entry: [VideoPackets,VidPackLen,NavPackets,NavPackLen]= sendAttVz(i,Active1,Roll,Pitch,Altitude,Yaw,i);
  state [VideoPackets,VidPackLen,NavPackets,NavPackLen] = sendAttVz(DataStamp_1,Active,Roll,Pitch,Altitude,Yaw,DataStamp_2) [function]
  (default) -> (junction 33)
  (junction 33) -> ModeSelector : {i = 1}
  ExecuteTrimCmd_State -> ModeSelector [order 1] : [mode~=4]
  ModeSelector -> ExecuteTrimCmd_State : [mode == 4]
      | {i=i+1;}
  ExecuteTrimCmd_State -> WakeUpNavVideo_State [order 2] : after(3,sec)
      | {i=i+1;}
  RunMotor6 -> ModeSelector : after(1,sec)
  WakeUpNavVideo_State -> StartNavDemo_State : after(1,sec)
      | {i = i +1;}
  StartNavDemo_State -> SetVideoChannel_State : after(0.1,sec)
      | {i=i+1;}
  SetVideoChannel_State -> BeginHover_State : after(0.1,sec)
      | {i =i +1;}
  BeginHover_State -> Control_State : after(1,sec)
      | {i=i+2;}
  Control_State -> RunMotor6 [order 1] : [mode~=4]
      | {i=i+1;}
  Control_State -> Control_State [order 2] : after(0.04,sec)
      | {i = i+2;}
  data: DataStamp function_input; DataStamp function_input; DataStamp function_input; DataStamp function_input; DataStamp function_input; In1 function_input; DataStamp_1 function_input; Active function_input; Roll function_input; Pitch function_input; Altitude function_input; Yaw function_input; DataStamp_2 function_input; VideoPackets function_output; VidPackLen function_output uint16; NavPackets function_output; NavPackLen function_output; Roll input double; Pitch input double; Altitude input double; Yaw input double; mode input; i local double; NavPackets output uint8 size=[500,1]; NavPackLen output double; VideoPackets output uint8 size=[40000,1]; VidPackLen output uint16; ErrorFlag output double; Active1 input double

== matlab function joystick_control/Ball Tracking/DIM Leds 9.2 to 9 Volts ==
  data: img_in input; bw_Green output
function bw_Green     = greenThreshold(img_in)
% justRed = (3*r-g-b);
% 
% 
% r = img_in(:,:,1);
% g = img_in(:,:,2);
% b = img_in(:,:,3);
% justGreen = (3*g-2*r-2*b);
% bw_Green = ~(0.9 > justGreen);


% r = img_in(:,:,1);
% g = img_in(:,:,2);
% b = img_in(:,:,3);
% justGreen = (3*g-1*r-2*b);
% bw_Green = ~(0.9 > justGreen);

% for MIT
r = img_in(:,:,1);
g = img_in(:,:,2);
b = img_in(:,:,3);
justGreen = (3*g-2*r-2*b);
bw_Green = ~(0.9 > justGreen);


% bw_Green = (g>0.6 & r<0.4 & b <0.4);
